simulink model "Gera_dados_local_PLMS_2015a"  (R2015a)
settings: Solver=ode4  StartTime=0.0  StopTime=120  FixedStep=0.005  RelTol=1e-3
settings Model: Creator=Fabricio  LastModifiedBy=Fabricio
settings DataIOCC: SignalLoggingSaveFormat=ModelDataLogs
settings OptimizationCC: ExpressionDepthLimit=2147483647  InitFltsAndDblsToZero=on
settings DebuggingCC: UnderspecifiedInitializationDetection=Classic  MergeDetectMultiDrivingBlocksExec=none  SolverPrmCheckMsg=warning  FcnCallInpInsideContextMsg=EnableAllAsWarning  StateNameClashWarn=warning
settings GRTTargetCC: CombineOutputUpdateFcns=off  GRTInterface=on

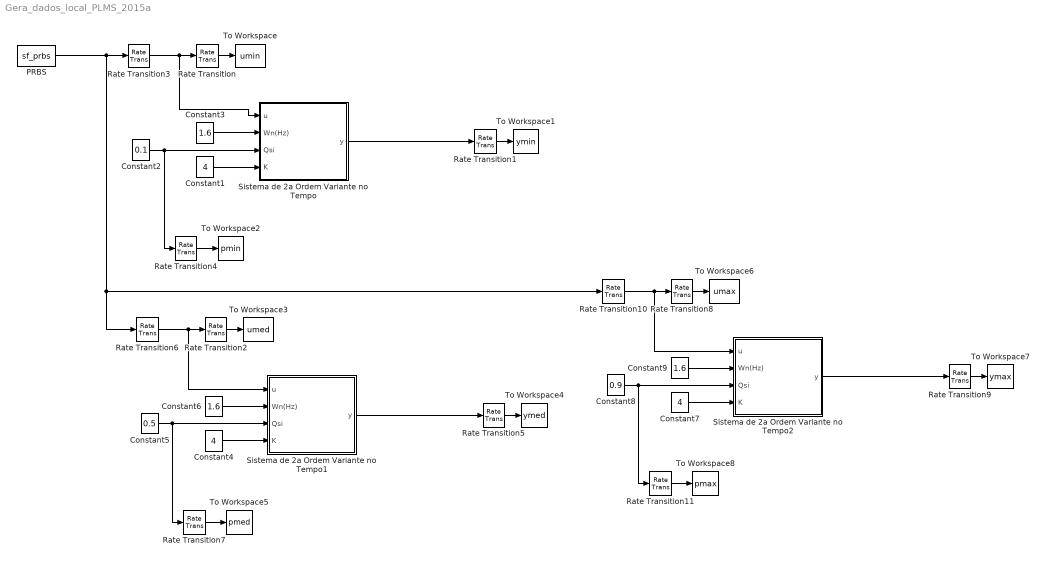
== system Gera_dados_local_PLMS_2015a ==
  Constant1 : Constant  Value=4
  Constant2 : Constant  Value=0.1
  Constant3 : Constant  Value=1.6
  Constant4 : Constant  Value=4
  Constant5 : Constant  Value=0.5
  Constant6 : Constant  Value=1.6
  Constant7 : Constant  Value=4
  Constant8 : Constant  Value=0.9
  Constant9 : Constant  Value=1.6
  PRBS : S-Function  FunctionName=sf_prbs  Parameters=K,N,Ts  SFunctionDeploymentMode=off  EnableBusSupport=off  mask{K=0.1, N=10, Ts=0.8}
      mask prompts: K "Ganho (K):"; N "Número de Células (usar 5, 7 ou 10):"; Ts "Tempo de amostragem (seg):"
      mask Display: disp('P R B S')
  Rate Transition{,1..3,5..6,8..10} (9 alike) : RateTransition
  Rate Transition11 : RateTransition  X0=0.05
  Rate Transition4 : RateTransition  X0=0.05
  Rate Transition7 : RateTransition  X0=0.05
  Sistema de 2a Ordem Variante no Tempo : Subsystem
  Sistema de 2a Ordem Variante no Tempo1 : Subsystem
  Sistema de 2a Ordem Variante no Tempo2 : Subsystem
  To Workspace : ToWorkspace  VariableName=umin  SampleTime=0.05
  To Workspace1 : ToWorkspace  VariableName=ymin  SampleTime=0.05
  To Workspace2 : ToWorkspace  VariableName=pmin  SampleTime=0.05
  To Workspace3 : ToWorkspace  VariableName=umed  SampleTime=0.05
  To Workspace4 : ToWorkspace  VariableName=ymed  SampleTime=0.05
  To Workspace5 : ToWorkspace  VariableName=pmed  SampleTime=0.05
  To Workspace6 : ToWorkspace  VariableName=umax  SampleTime=0.05
  To Workspace7 : ToWorkspace  VariableName=ymax  SampleTime=0.05
  To Workspace8 : ToWorkspace  VariableName=pmax  SampleTime=0.05
  wires:
  Rate Transition/1 -> To Workspace/1
  Rate Transition1/1 -> To Workspace1/1
  Constant3/1 -> Sistema de 2a Ordem Variante no Tempo/2(Wn(Hz))
  Rate Transition3/1 -> Rate Transition/1, Sistema de 2a Ordem Variante no Tempo/1(u)
  Rate Transition4/1 -> To Workspace2/1
  Constant2/1 -> Rate Transition4/1, Sistema de 2a Ordem Variante no Tempo/3(Qsi)
  Constant1/1 -> Sistema de 2a Ordem Variante no Tempo/4(K)
  Constant5/1 -> Rate Transition7/1, Sistema de 2a Ordem Variante no Tempo1/3(Qsi)
  Rate Transition2/1 -> To Workspace3/1
  Constant4/1 -> Sistema de 2a Ordem Variante no Tempo1/4(K)
  Rate Transition7/1 -> To Workspace5/1
  Constant6/1 -> Sistema de 2a Ordem Variante no Tempo1/2(Wn(Hz))
  Rate Transition5/1 -> To Workspace4/1
  Rate Transition6/1 -> Rate Transition2/1, Sistema de 2a Ordem Variante no Tempo1/1(u)
  Constant8/1 -> Rate Transition11/1, Sistema de 2a Ordem Variante no Tempo2/3(Qsi)
  Rate Transition8/1 -> To Workspace6/1
  Constant7/1 -> Sistema de 2a Ordem Variante no Tempo2/4(K)
  Rate Transition11/1 -> To Workspace8/1
  Constant9/1 -> Sistema de 2a Ordem Variante no Tempo2/2(Wn(Hz))
  Rate Transition9/1 -> To Workspace7/1
  PRBS/1 -> Rate Transition10/1, Rate Transition6/1, Rate Transition3/1
  Rate Transition10/1 -> Rate Transition8/1, Sistema de 2a Ordem Variante no Tempo2/1(u)
  Sistema de 2a Ordem Variante no Tempo/1(y) -> Rate Transition1/1
  Sistema de 2a Ordem Variante no Tempo1/1(y) -> Rate Transition5/1
  Sistema de 2a Ordem Variante no Tempo2/1(y) -> Rate Transition9/1

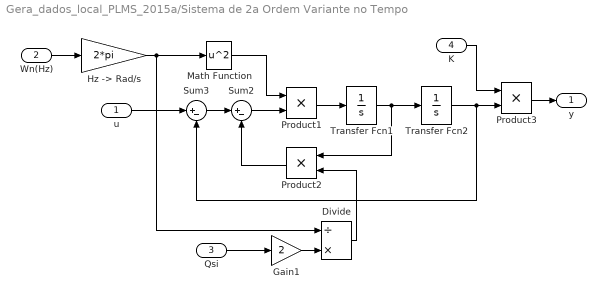
== system Gera_dados_local_PLMS_2015a/Sistema de 2a Ordem Variante no Tempo ==
  u : Inport
  Wn(Hz) : Inport  Port=2
  Qsi : Inport  Port=3
  K : Inport  Port=4
  Divide : Product  Inputs=/*
  Gain1 : Gain  Gain=2
  "Hz -> Rad/s" : Gain  Gain=2*pi
  Math Function : Math  Operator=square  SaturateOnIntegerOverflow=on
  Product1 : Product  RndMeth=Zero
  Product2 : Product  RndMeth=Zero
  Product3 : Product  RndMeth=Zero
  Sum2 : Sum  Inputs=|+-
  Sum3 : Sum  Inputs=|+-
  Transfer Fcn1 : TransferFcn  Denominator=[1 0]
  Transfer Fcn2 : TransferFcn  Denominator=[1 0]
  y : Outport
  wires:
  Product1/1 -> Transfer Fcn1/1
  Sum2/1 -> Product1/2
  Product2/1 -> Sum2/2
  Transfer Fcn1/1 -> Product2/1, Transfer Fcn2/1
  Sum3/1 -> Sum2/1
  Transfer Fcn2/1 -> Sum3/2, Product3/2
  Wn(Hz)/1 -> "Hz -> Rad/s"/1
  Math Function/1 -> Product1/1
  Qsi/1 -> Gain1/1
  Gain1/1 -> Divide/2
  Divide/1 -> Product2/2
  u/1 -> Sum3/1
  K/1 -> Product3/1
  Product3/1 -> y/1
  "Hz -> Rad/s"/1 -> Math Function/1, Divide/1

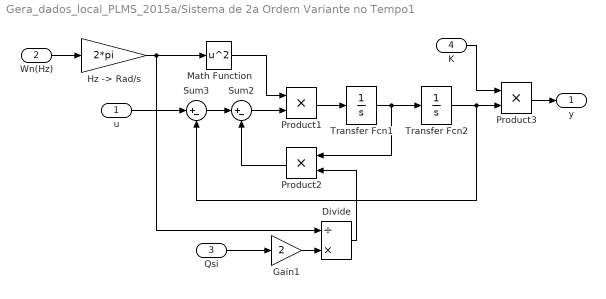
== system Gera_dados_local_PLMS_2015a/Sistema de 2a Ordem Variante no Tempo1 ==
  u : Inport
  Wn(Hz) : Inport  Port=2
  Qsi : Inport  Port=3
  K : Inport  Port=4
  Divide : Product  Inputs=/*
  Gain1 : Gain  Gain=2
  "Hz -> Rad/s" : Gain  Gain=2*pi
  Math Function : Math  Operator=square  SaturateOnIntegerOverflow=on
  Product1 : Product  RndMeth=Zero
  Product2 : Product  RndMeth=Zero
  Product3 : Product  RndMeth=Zero
  Sum2 : Sum  Inputs=|+-
  Sum3 : Sum  Inputs=|+-
  Transfer Fcn1 : TransferFcn  Denominator=[1 0]
  Transfer Fcn2 : TransferFcn  Denominator=[1 0]
  y : Outport
  wires:
  Product1/1 -> Transfer Fcn1/1
  Sum2/1 -> Product1/2
  Product2/1 -> Sum2/2
  Transfer Fcn1/1 -> Product2/1, Transfer Fcn2/1
  Sum3/1 -> Sum2/1
  Transfer Fcn2/1 -> Sum3/2, Product3/2
  Wn(Hz)/1 -> "Hz -> Rad/s"/1
  Math Function/1 -> Product1/1
  Qsi/1 -> Gain1/1
  Gain1/1 -> Divide/2
  Divide/1 -> Product2/2
  u/1 -> Sum3/1
  K/1 -> Product3/1
  Product3/1 -> y/1
  "Hz -> Rad/s"/1 -> Math Function/1, Divide/1

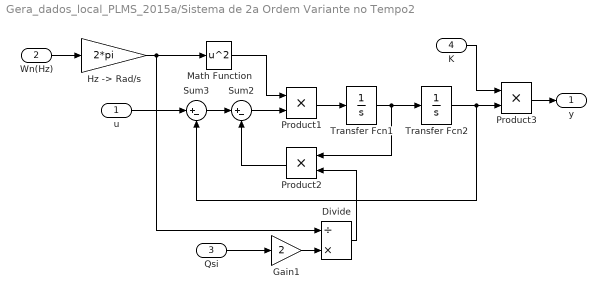
== system Gera_dados_local_PLMS_2015a/Sistema de 2a Ordem Variante no Tempo2 ==
  u : Inport
  Wn(Hz) : Inport  Port=2
  Qsi : Inport  Port=3
  K : Inport  Port=4
  Divide : Product  Inputs=/*
  Gain1 : Gain  Gain=2
  "Hz -> Rad/s" : Gain  Gain=2*pi
  Math Function : Math  Operator=square  SaturateOnIntegerOverflow=on
  Product1 : Product  RndMeth=Zero
  Product2 : Product  RndMeth=Zero
  Product3 : Product  RndMeth=Zero
  Sum2 : Sum  Inputs=|+-
  Sum3 : Sum  Inputs=|+-
  Transfer Fcn1 : TransferFcn  Denominator=[1 0]
  Transfer Fcn2 : TransferFcn  Denominator=[1 0]
  y : Outport
  wires:
  Product1/1 -> Transfer Fcn1/1
  Sum2/1 -> Product1/2
  Product2/1 -> Sum2/2
  Transfer Fcn1/1 -> Product2/1, Transfer Fcn2/1
  Sum3/1 -> Sum2/1
  Transfer Fcn2/1 -> Sum3/2, Product3/2
  Wn(Hz)/1 -> "Hz -> Rad/s"/1
  Math Function/1 -> Product1/1
  Qsi/1 -> Gain1/1
  Gain1/1 -> Divide/2
  Divide/1 -> Product2/2
  u/1 -> Sum3/1
  K/1 -> Product3/1
  Product3/1 -> y/1
  "Hz -> Rad/s"/1 -> Math Function/1, Divide/1
